simulink model "LIM_FOC_RNN_PID_1"  (R2021b)
settings: Solver=VariableStepAuto  StartTime=0.0  StopTime=3  RelTol=1e-3
values from neighbouring files (symbols this model uses):
  a1 = 1    [parameters_FOC.m]
  a2 = 1    [parameters_FOC.m]
  a3 = 1    [parameters_FOC.m]
  a4 = 1    [parameters_FOC.m]
  b1 = 1    [parameters_FOC.m]
  b2 = 1    [parameters_FOC.m]
  b3 = 1    [parameters_FOC.m]
  b4 = 1    [parameters_FOC.m]
  D = 0.25    [FOC_parameters_Basil.m]    (also in parameters_FOC.m)
  Llr = 0.005    [parameters_FOC.m]
  Lls = 0.005    [parameters_FOC.m]
  Lm = 0.0416    [FOC_parameters_Basil.m]    (also in parameters_FOC.m = 0.4)
  M = 4.775    [FOC_parameters_Basil.m]    (also in parameters_FOC.m)
  P = 2    [FOC_parameters_Basil.m]    (also in parameters_FOC.m = 4)
  ql = 1    [parameters_FOC.m]
  qq1 = 1    [parameters_FOC.m]
  qq2 = 1    [parameters_FOC.m]
  qq3 = 1    [parameters_FOC.m]
  qq4 = 1    [parameters_FOC.m]
  Rr = 11.78    [parameters_FOC.m]
  Rs = 13.2    [parameters_FOC.m]
  w1 = 1    [parameters_FOC.m]
  w2 = 1    [parameters_FOC.m]
  w3 = 1    [parameters_FOC.m]
  w4 = 1    [parameters_FOC.m]
libraries: neural x12, spsMosfetLib x6, slpidlib x3, spsVoltageMeasurementLib x3, simulink_extras x1, spsDCVoltageSourceLib x1, spsGroundLib x1, spspowerguiLib x1
settings Model: Creator=Hassan Alam  LastModifiedBy=Basilisk
settings SolverCC: ZeroCrossAlgorithm=Adaptive  AlgebraicLoopSolver=TrustRegion
settings DebuggingCC: MaskedZcDiagnostic=none  IgnoredZcDiagnostic=none  SFMachineParentedDataDiag=warning  ArithmeticOperatorsInVariantConditions=warning
settings SFSimCC: CustomCodeUndefinedFunction=UseInterfaceOnly

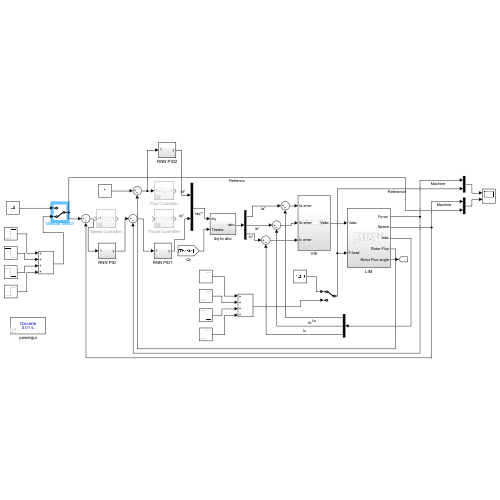
[thumbnail: Simulink's stored preview of the top-level diagram]
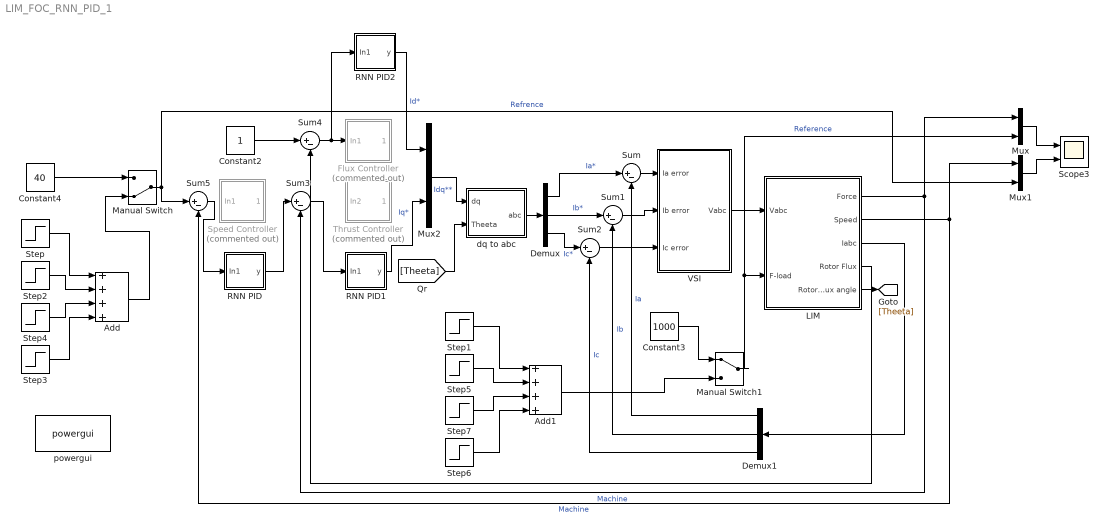
== system LIM_FOC_RNN_PID_1 ==
  Add : Sum  Inputs=++++
  Add1 : Sum  Inputs=++++
  Constant2 : Constant
  Constant3 : Constant  Value=1000
  Constant4 : Constant  Value=40
  Demux : Demux  Outputs=3
  Demux1 : Demux  Outputs=3
  Flux Controller : Subsystem  Commented=on
  LIM : Subsystem
  Manual Switch : ManualSwitch  CurrentSetting=0
  Manual Switch1 : ManualSwitch
  Mux : Mux  Inputs=2
  Mux1 : Mux  Inputs=2
  Mux2 : Mux  Inputs=2
  RNN PID : Subsystem
  RNN PID1 : Subsystem
  RNN PID2 : Subsystem
  Scope3 : Scope  NumInputPorts=2
  Speed Controller : Subsystem  Commented=on
  Step : Step  Time=0.5  Before=1  After=1.6  SampleTime=0
  Step1 : Step  Time=0.5  After=4  SampleTime=0
  Step2 : Step  Time=0.9  After=-0.4  SampleTime=0
  Step3 : Step  Time=2  After=0.5  SampleTime=0
  Step4 : Step  Time=1.5  After=-0.7  SampleTime=0
  Step5 : Step  Time=0.9  After=5  SampleTime=0
  Step6 : Step  Time=2  After=3  SampleTime=0
  Step7 : Step  Time=1.5  After=-2  SampleTime=0
  Sum{,1..5} (6 alike) : Sum  Inputs=|+-
  Thrust Controller : Subsystem  Commented=on
  VSI : Subsystem
  dq to abc : Subsystem
  powergui : spspowerguiLib/powergui  Priority=1  SimulationMode=Discrete  SampleTime=0.01  frequency=60  Iterations=50  frequencyindice=0  Pbase=100e6  ErrMax=1e-4  UnitsV=kV  UnitsW=MW  buscounter=0  FunctionMessages=off  echomessages=off  EnableUseOfTLC=off  CurrentSourceSwitches=off  DisableSnubberDevices=off  DisableRonSwitches=off  DisableVfSwitches=off  DisplayEquations=off  AutomaticDiscreteSolvers=off  SolverType=Tustin/Backward Euler (TBE)  Interpol=off  ExternalGateDelay=off  methode=off  Ts=100  x0status=blocks  SPID=on  SwTol=0  HookPort=off  NonlinearTolerance=1e-4  nMaxIteration=100  ContinueOnMaxIteration=off  RestoreLinks=warning  ResistiveCurrentMeasurement=off  Frange=[0:2:500]  Ylog=off  Xlog=on  ShowGrid=off  save=off  variable=ZData  structure=0  ZoomFFT=off  StartTime=0.0  cycles=1  DisplayStyle=1  fundamental=60  FreqAxis=off  MaxFrequency=1000  frequencyindicesteady=1  RmsSteady=1  display=off
  wires:
  Sum2/1 -> VSI/3(Ic error)
  Sum1/1 -> VSI/2(Ib error)
  Sum/1 -> VSI/1(Ia error)
  dq to abc/1(abc) -> Demux/1
  Demux/2 -> Sum1/1  "Ib*"
  Demux/1 -> Sum/1  "Ia*"
  Demux/3 -> Sum2/1  "Ic*"
  RNN PID1/1(y) -> Mux2/2  "Iq*"
  RNN PID2/1(y) -> Mux2/1  "Id*"
  Mux2/1 -> dq to abc/1(dq)  "Idq**"
  Demux1/1 -> Sum/2  "Ia"
  Demux1/2 -> Sum1/2  "Ib"
  Demux1/3 -> Sum2/2  "Ic"
  LIM/2(" Speed") -> Mux1/1, Sum5/2  "Machine"
  Constant2/1 -> Sum4/1
  Sum4/1 -> RNN PID2/1(In1), Flux Controller/1(In1)
  LIM/4(" Rotor Flux") -> Sum4/2
  [Theeta] -> dq to abc/2(Theeta)
  Constant4/1 -> Manual Switch/1
  VSI/1(Vabc) -> LIM/1(Vabc)
  Sum5/1 -> RNN PID/1(In1)
  LIM/5(" Rotor Flux angle") -> [Theeta]
  LIM/3(" Iabc") -> Demux1/1
  Sum3/1 -> RNN PID1/1(In1)
  Step/1 -> Add/1
  Constant3/1 -> Manual Switch1/1
  Manual Switch1/1 -> LIM/2(F-load), Mux/2  "Reference"
  Add1/1 -> Manual Switch1/2
  Manual Switch/1 -> Sum5/1, Mux1/2  "Refrence"
  Mux/1 -> Scope3/1
  Mux1/1 -> Scope3/2
  LIM/1("Force ") -> Mux/1, Sum3/2  "Machine"
  RNN PID/1(y) -> Sum3/1
  Step2/1 -> Add/2
  Step3/1 -> Add/4
  Step4/1 -> Add/3
  Add/1 -> Manual Switch/2
  Step7/1 -> Add1/3
  Step6/1 -> Add1/4
  Step5/1 -> Add1/2
  Step1/1 -> Add1/1

== system LIM_FOC_RNN_PID_1/Flux Controller ==
  In1 : Inport
  Gain2 : Gain  Gain=6000
  Gain3 : Gain  Gain=0.001
  Integrator : Integrator
  Sum2 : Sum
  Out1 : Outport
  wires:
  In1/1 -> Gain3/1, Gain2/1
  Gain3/1 -> Integrator/1
  Gain2/1 -> Sum2/1
  Integrator/1 -> Sum2/2
  Sum2/1 -> Out1/1

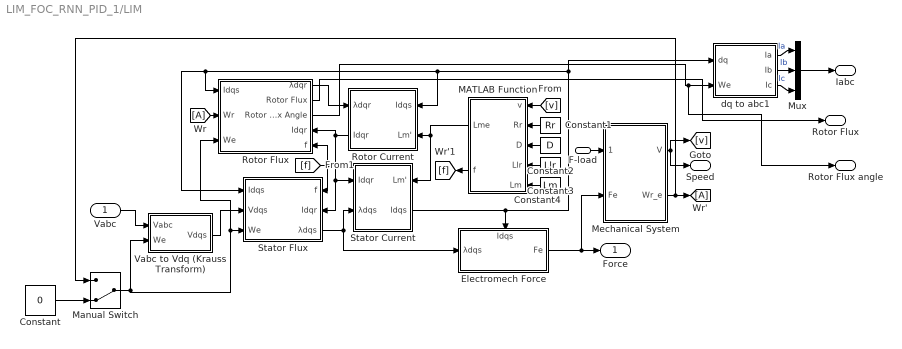
== system LIM_FOC_RNN_PID_1/LIM ==
  Vabc : Inport
  F-load : Inport  Port=2
  Constant : Constant  Value=0
  Constant1 : Constant  Value=Rr
  Constant2 : Constant  Value=D
  Constant3 : Constant  Value=Llr
  Constant4 : Constant  Value=Lm
  Electromech Force : Subsystem
      settings: PortSchema="{\"entries\":[{\"content\":{\"sides\":[{\"content\":{\"connectorIds\":[\"In1\"]},\"type\":\"ConnectorPlacement.EquallySpacedRectSide\",\"uuid\":\"a4b29cca-9cb0-4324-9244-2049ffc93668\"},{\"content\":{\"connectorIds\":[\"Out1\"],\"side\":\"RIGHT\"},\"type\":\"ConnectorPlacement.EquallySpacedRectSide\",\"uuid\":\"b20ff3ac-d40e-4f59-bb91-f6f2c0c6ca63\"},{\"content\":{\"connectorIds\":[\"In2\"],\"side\":\"TOP\"},\"type\":\"ConnectorPlacement.EquallySpacedRectSide\",\"uuid\":\"55342d43-b8f9-4aa9-846c-26670e92f4ca\"},{\"content\":{\"connectorIds\":[],\"side\":\"HIDDEN\"},\"type\":\"ConnectorPlacement.EquallySpacedRectSide\",\"uuid\":\"5fed22a0-a45a-430c-a997-0be85a9315bb\"}]},\"type\":\"ConnectorPlacement.EquallySpacedConnector\",\"uuid\":\"78d5652d-2b6b-4c50-974b-d09ad892483f\"}],\"packageUris\":[\"http://schema.mathworks.com/mf0/Connector/R2020b\"],\"version\":\"1.0\"}"
  MATLAB Function : MATLAB Function  TreatAsAtomicUnit=on
  Manual Switch : ManualSwitch  CurrentSetting=0
  Mechanical System : Subsystem
  Mux : Mux  Inputs=3
  Rotor Current : Subsystem
      settings: PortSchema="{\"entries\":[{\"content\":{\"sides\":[{\"content\":{\"connectorIds\":[\"In1\",\"Out1\"]},\"type\":\"ConnectorPlacement.EquallySpacedRectSide\",\"uuid\":\"b9a9f404-9b3b-4182-a50e-1bf7cef191e8\"},{\"content\":{\"connectorIds\":[\"In2\",\"In3\"],\"side\":\"RIGHT\"},\"type\":\"ConnectorPlacement.EquallySpacedRectSide\",\"uuid\":\"68159d79-7975-4fd0-98a3-7e35432781a2\"},{\"content\":{\"connectorIds\":[],\"side\":\"TOP\"},\"type\":\"ConnectorPlacement.EquallySpacedRectSide\",\"uuid\":\"0c4dbb5d-b4d4-4876-b829-49090bd6eeb8\"},{\"content\":{\"connectorIds\":[],\"side\":\"BOTTOM\"},\"type\":\"ConnectorPlacement.EquallySpacedRectSide\",\"uuid\":\"e42509db-2e5f-42f8-9a91-9046ba95e836\"},{\"content\":{\"connectorIds\":[],\"side\":\"HIDDEN\"},\"type\":\"ConnectorPlacement.EquallySpacedRectSide\",\"uuid\":\"f2a65973-682a-4dd6-b429-3fa72198cae4\"}]},\"type\":\"ConnectorPlacement.EquallySpacedConnector\",\"uuid\":\"744eb17f-cf6a-4151-90db-78263b57d619\"}],\"packageUris\":[\"http://schema.mathworks.com/mf0/Connector/R2020b\"],\"version\":\"1.0\"}"
  Rotor Flux : Subsystem
      settings: PortSchema="{\"entries\":[{\"content\":{\"sides\":[{\"content\":{\"connectorIds\":[\"In1\",\"In2\",\"In3\"]},\"type\":\"ConnectorPlacement.EquallySpacedRectSide\",\"uuid\":\"b9a9f404-9b3b-4182-a50e-1bf7cef191e8\"},{\"content\":{\"connectorIds\":[\"Out1\",\"Out2\",\"Out3\",\"In4\",\"In5\"],\"side\":\"RIGHT\"},\"type\":\"ConnectorPlacement.EquallySpacedRectSide\",\"uuid\":\"68159d79-7975-4fd0-98a3-7e35432781a2\"},{\"content\":{\"connectorIds\":[],\"side\":\"TOP\"},\"type\":\"ConnectorPlacement.EquallySpacedRectSide\",\"uuid\":\"0c4dbb5d-b4d4-4876-b829-49090bd6eeb8\"},{\"content\":{\"connectorIds\":[],\"side\":\"HIDDEN\"},\"type\":\"ConnectorPlacement.EquallySpacedRectSide\",\"uuid\":\"f2a65973-682a-4dd6-b429-3fa72198cae4\"}]},\"type\":\"ConnectorPlacement.EquallySpacedConnector\",\"uuid\":\"744eb17f-cf6a-4151-90db-78263b57d619\"}],\"packageUris\":[\"http://schema.mathworks.com/mf0/Connector/R2020b\"],\"version\":\"1.0\"}"
  Stator Current : Subsystem
      settings: PortSchema="{\"entries\":[{\"content\":{\"sides\":[{\"content\":{\"connectorIds\":[\"In1\",\"In2\"]},\"type\":\"ConnectorPlacement.EquallySpacedRectSide\",\"uuid\":\"c6a8d684-b7d2-4173-9e8a-0a77b360fa3b\"},{\"content\":{\"connectorIds\":[\"In3\",\"Out1\"],\"side\":\"RIGHT\"},\"type\":\"ConnectorPlacement.EquallySpacedRectSide\",\"uuid\":\"6b547613-238c-47a7-9a25-113e0bcf67e8\"},{\"content\":{\"connectorIds\":[],\"side\":\"TOP\"},\"type\":\"ConnectorPlacement.EquallySpacedRectSide\",\"uuid\":\"9eb731ca-d22d-4bff-90d4-9f452150afc4\"},{\"content\":{\"connectorIds\":[],\"side\":\"HIDDEN\"},\"type\":\"ConnectorPlacement.EquallySpacedRectSide\",\"uuid\":\"3386087c-4273-46bf-b0bc-9959c9fde15b\"}]},\"type\":\"ConnectorPlacement.EquallySpacedConnector\",\"uuid\":\"3fded039-aa6e-4722-8a98-01f4cd5eabc0\"}],\"packageUris\":[\"http://schema.mathworks.com/mf0/Connector/R2020b\"],\"version\":\"1.0\"}"
  Stator Flux : Subsystem
      settings: PortSchema="{\"entries\":[{\"content\":{\"sides\":[{\"content\":{\"connectorIds\":[\"In1\",\"In2\",\"In3\"]},\"type\":\"ConnectorPlacement.EquallySpacedRectSide\",\"uuid\":\"a4b29cca-9cb0-4324-9244-2049ffc93668\"},{\"content\":{\"connectorIds\":[\"In4\",\"In5\",\"Out1\"],\"side\":\"RIGHT\"},\"type\":\"ConnectorPlacement.EquallySpacedRectSide\",\"uuid\":\"b20ff3ac-d40e-4f59-bb91-f6f2c0c6ca63\"},{\"content\":{\"connectorIds\":[],\"side\":\"TOP\"},\"type\":\"ConnectorPlacement.EquallySpacedRectSide\",\"uuid\":\"55342d43-b8f9-4aa9-846c-26670e92f4ca\"},{\"content\":{\"connectorIds\":[],\"side\":\"HIDDEN\"},\"type\":\"ConnectorPlacement.EquallySpacedRectSide\",\"uuid\":\"5fed22a0-a45a-430c-a997-0be85a9315bb\"}]},\"type\":\"ConnectorPlacement.EquallySpacedConnector\",\"uuid\":\"78d5652d-2b6b-4c50-974b-d09ad892483f\"}],\"packageUris\":[\"http://schema.mathworks.com/mf0/Connector/R2020b\"],\"version\":\"1.0\"}"
  Vabc to Vdq (Krauss Transform) : Subsystem
  dq to abc1 : Subsystem
  "Force " : Outport
  " Speed" : Outport  Port=2
  " Iabc" : Outport  Port=3
  " Rotor Flux" : Outport  Port=4
  " Rotor Flux angle" : Outport  Port=5
  wires:
  Electromech Force/1(Fe) -> Mechanical System/2(Fe), "Force "/1
  F-load/1 -> Mechanical System/1(F-load)
  Mechanical System/1(V) -> " Speed"/1, [v]
  Stator Flux/1(λdqs) -> Stator Current/2(λdqs), Electromech Force/1(λdqs)
  Stator Current/1(Idqs) -> Electromech Force/2(Idqs), dq to abc1/1(dq), Rotor Flux/1(Idqs), Stator Flux/1(Idqs), Rotor Current/2(Idqs)
  Rotor Flux/1(λdqr) -> Rotor Current/1(λdqr)
  Rotor Current/1(Idqr) -> Rotor Flux/4(Idqr), Stator Flux/5(Idqr), Stator Current/1(Idqr)
  [A] -> Rotor Flux/2(Wr)
  Vabc/1 -> Vabc to Vdq (Krauss Transform)/1(Vabc)
  Vabc to Vdq (Krauss Transform)/1(Vdqs) -> Stator Flux/2(Vdqs)
  MATLAB Function/1(Lme) -> Stator Current/3(Lm'), Rotor Current/3(Lm')
  [v] -> MATLAB Function/1(v)
  Constant1/1 -> MATLAB Function/2(Rr)
  Constant2/1 -> MATLAB Function/3(D)
  Constant3/1 -> MATLAB Function/4(Llr)
  Constant4/1 -> MATLAB Function/5(Lm)
  MATLAB Function/2(f) -> [f]
  [f] -> Rotor Flux/5(f), Stator Flux/4(f)
  Mechanical System/2(Wr_e) -> Manual Switch/1, [A]
  Manual Switch/1 -> Vabc to Vdq (Krauss Transform)/2(We), Rotor Flux/3(We), Stator Flux/3(We)
  Constant/1 -> Manual Switch/2
  Mux/1 -> " Iabc"/1
  dq to abc1/2(Ib) -> Mux/2  "Ib"
  dq to abc1/3(Ic) -> Mux/3  "Ic"
  dq to abc1/1(Ia) -> Mux/1  "Ia"
  Rotor Flux/2(Rotor Flux) -> " Rotor Flux"/1
  Rotor Flux/3(Rotor Flux Angle) -> " Rotor Flux angle"/1, dq to abc1/2(We)

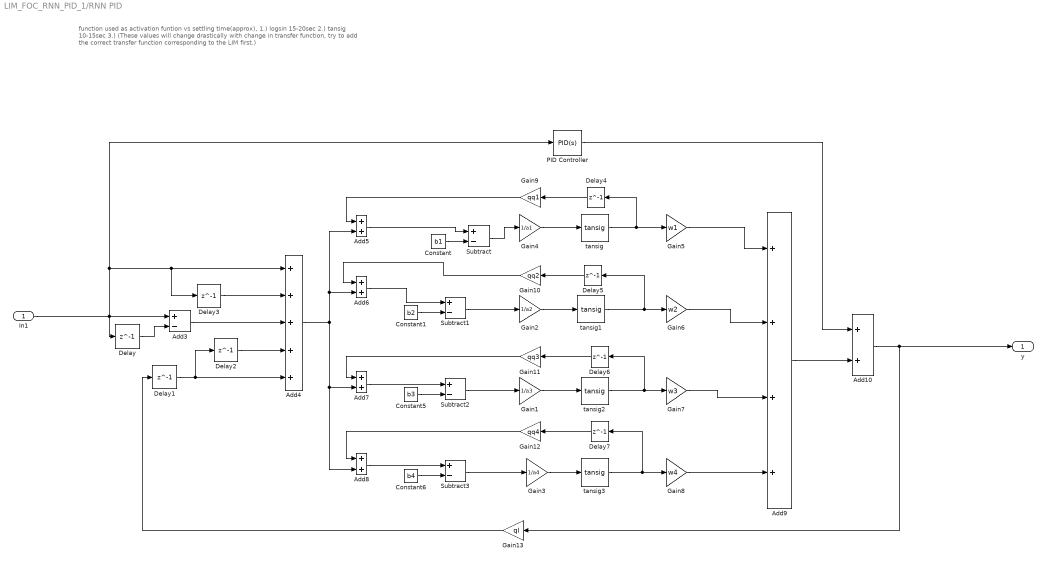
== system LIM_FOC_RNN_PID_1/RNN PID ==
  note: function used as activation funtion vs settling time(approx),
      | 1.) logsin   15-20sec
      | 2.) tansig   10-15sec
      | 3.)
      | (These values will change drastically with change in transfer function, try to add the correct transfer function corresponding to the LIM first.)
  In1 : Inport
  Add{5..8,10} (5 alike) : Sum
  Add3 : Sum  Inputs=+-
  Add4 : Sum  Inputs=+++++
  Add9 : Sum  Inputs=++++
  Constant : Constant  Value=b1
  Constant1 : Constant  Value=b2
  Constant5 : Constant  Value=b3
  Constant6 : Constant  Value=b4
  Delay{,1..7} (8 alike) : Delay  DelayLength=1
  Gain1 : Gain  Gain=1/a3
  Gain10 : Gain  Gain=qq2
  Gain11 : Gain  Gain=qq3
  Gain12 : Gain  Gain=qq4
  Gain13 : Gain  Gain=ql
  Gain2 : Gain  Gain=1/a2
  Gain3 : Gain  Gain=1/a4
  Gain4 : Gain  Gain=1/a1
  Gain5 : Gain  Gain=w1
  Gain6 : Gain  Gain=w2
  Gain7 : Gain  Gain=w3
  Gain8 : Gain  Gain=w4
  Gain9 : Gain  Gain=qq1
  PID Controller : slpidlib/PID Controller  Controller=PID  Form=Parallel  TimeDomain=Continuous-time  UseExternalTs=off  SampleTime=-1  IntegratorMethod=Forward Euler  FilterMethod=Forward Euler  ControllerParametersSource=internal  P=10  I=100  D=10  UseFilter=on  N=100  TunerSelectOption=Transfer Function Based (PID Tuner App)  InitialConditionSource=internal  InitialConditionForIntegrator=0  InitialConditionForFilter=0  DifferentiatorICPrevScaledInput=0  ExternalReset=none  TrackingMode=off  Kt=1  LimitOutput=off  SatLimitsSource=internal  UpperSaturationLimit=inf  LowerSaturationLimit=-inf  LinearizeAsGain=on  AntiWindupMode=none  Kb=1  POutMin=[]  POutMax=[]  IOutMin=[]  IOutMax=[]  DOutMin=[]  DOutMax=[]  NOutMin=[]  NOutMax=[]  SumOutMin=[]  SumOutMax=[]  SaturationOutMin=[]  SaturationOutMax=[]  PParamMin=[]  PParamMax=[]  IParamMin=[]  IParamMax=[]  DParamMin=[]  DParamMax=[]  NParamMin=[]  NParamMax=[]  KbParamMin=[]  KbParamMax=[]  KtParamMin=[]  KtParamMax=[]  KbOutMin=[]  KbOutMax=[]  KtOutMin=[]  KtOutMax=[]  IntegratorOutMin=[]  IntegratorOutMax=[]  FilterOutMin=[]  FilterOutMax=[]  SumI1OutMin=[]  SumI1OutMax=[]  SumI2OutMin=[]  SumI2OutMax=[]  SumI3OutMin=[]  SumI3OutMax=[]  SumI4OutMin=[]  SumI4OutMax=[]  SumDOutMin=[]  SumDOutMax=[]  DifferentiatorOutMin=[]  DifferentiatorOutMax=[]  FilterDiffOutCoefMin=[]  FilterDiffOutCoefMax=[]  ReciprocalOutMin=[]  ReciprocalOutMax=[]  SumDenOutMin=[]  SumDenOutMax=[]  SumNumOutMin=[]  SumNumOutMax=[]  DivideOutMin=[]  DivideOutMax=[]  UdiffTsProdOutMin=[]  UdiffTsProdOutMax=[]  NTsProdOutMin=[]  NTsProdOutMax=[]  UintegralTsProdOutMin=[]  UintegralTsProdOutMax=[]  UngainTsProdOutMin=[]  UngainTsProdOutMax=[]  IntegratorContinuousStateAttributes=''  IntegratorStateMustResolveToSignalObject=off  IntegratorRTWStateStorageClass=Auto  FilterContinuousStateAttributes=''  FilterStateMustResolveToSignalObject=off  FilterRTWStateStorageClass=Auto  ParallelPVariant=InternalParameters  IdealPVariant=Disabled  IVariant=InternalParameters  DVariant=InternalParameters  IntegratorVariant=Continuous  SatVariant=Disabled  AWVariant=Passthrough  PCopyVariant=Disabled  TRVariant=Disabled  FdbkBlocksVariant=Forward  IdealPFdbkVariant=Disabled  SatFdbkVariant=Disabled  DerivativeFilterVariant=ContFilter  NVariant=InternalParameters  NCopyVariant=Disabled  FilterICVariant=InternalICsFilter  IntegratorICVariant=InternalICs  ExternalResetVariant=Disabled  TRSumVariant=Passthrough  SumFdbkVariant=Disabled  SumVariant=Sum_PID  TsampFilterVariant=InternalTs  TsampNgainVariant=Passthrough  TsampIntegralVariant=Passthrough  ExternalSaturationOutDataTypeStr=Inherit: Same as second input
  Subtract{,1..3} (4 alike) : Sum  Inputs=+-
  tansig{,1..3} (4 alike) : neural/Transfer Functions/tansig
  y : Outport
  wires:
  Gain11/1 -> Add7/1
  Delay6/1 -> Gain11/1
  Constant5/1 -> Subtract2/2
  Gain8/1 -> Add9/4
  tansig1/1 -> Delay5/1, Gain6/1
  Gain1/1 -> tansig2/1
  tansig3/1 -> Delay7/1, Gain8/1
  Gain12/1 -> Add8/1
  Add10/1 -> y/1, Gain13/1
  Add3/1 -> Add4/3
  Delay/1 -> Add3/2
  Constant/1 -> Subtract/2
  Delay1/1 -> Delay2/1, Add4/5
  Add9/1 -> Add10/2
  Add5/1 -> Subtract/1
  Gain6/1 -> Add9/2
  Delay7/1 -> Gain12/1
  Subtract2/1 -> Gain1/1
  Gain7/1 -> Add9/3
  tansig2/1 -> Delay6/1, Gain7/1
  tansig/1 -> Delay4/1, Gain5/1
  Add4/1 -> Add8/2, Add7/2, Add6/2, Add5/2
  Gain5/1 -> Add9/1
  In1/1 -> PID Controller/1, Delay3/1, Add4/1, Add3/1, Delay/1
  Subtract3/1 -> Gain3/1
  Delay4/1 -> Gain9/1
  Gain4/1 -> tansig/1
  Add8/1 -> Subtract3/1
  Subtract/1 -> Gain4/1
  PID Controller/1 -> Add10/1
  Constant1/1 -> Subtract1/2
  Gain10/1 -> Add6/1
  Gain13/1 -> Delay1/1
  Gain9/1 -> Add5/1
  Constant6/1 -> Subtract3/2
  Delay2/1 -> Add4/4
  Add6/1 -> Subtract1/1
  Gain3/1 -> tansig3/1
  Gain2/1 -> tansig1/1
  Subtract1/1 -> Gain2/1
  Add7/1 -> Subtract2/1
  Delay3/1 -> Add4/2
  Delay5/1 -> Gain10/1

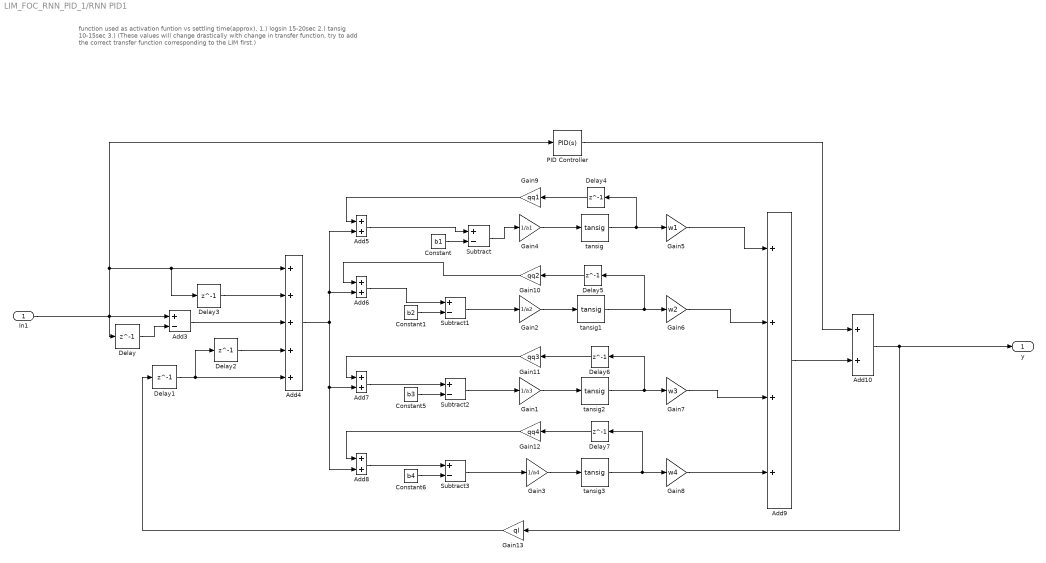
== system LIM_FOC_RNN_PID_1/RNN PID1 ==
  note: function used as activation funtion vs settling time(approx),
      | 1.) logsin   15-20sec
      | 2.) tansig   10-15sec
      | 3.)
      | (These values will change drastically with change in transfer function, try to add the correct transfer function corresponding to the LIM first.)
  In1 : Inport
  Add{5..8,10} (5 alike) : Sum
  Add3 : Sum  Inputs=+-
  Add4 : Sum  Inputs=+++++
  Add9 : Sum  Inputs=++++
  Constant : Constant  Value=b1
  Constant1 : Constant  Value=b2
  Constant5 : Constant  Value=b3
  Constant6 : Constant  Value=b4
  Delay{,1..7} (8 alike) : Delay  DelayLength=1
  Gain1 : Gain  Gain=1/a3
  Gain10 : Gain  Gain=qq2
  Gain11 : Gain  Gain=qq3
  Gain12 : Gain  Gain=qq4
  Gain13 : Gain  Gain=ql
  Gain2 : Gain  Gain=1/a2
  Gain3 : Gain  Gain=1/a4
  Gain4 : Gain  Gain=1/a1
  Gain5 : Gain  Gain=w1
  Gain6 : Gain  Gain=w2
  Gain7 : Gain  Gain=w3
  Gain8 : Gain  Gain=w4
  Gain9 : Gain  Gain=qq1
  PID Controller : slpidlib/PID Controller  Controller=PID  Form=Parallel  TimeDomain=Continuous-time  UseExternalTs=off  SampleTime=-1  IntegratorMethod=Forward Euler  FilterMethod=Forward Euler  ControllerParametersSource=internal  P=10  I=100  D=10  UseFilter=on  N=100  TunerSelectOption=Transfer Function Based (PID Tuner App)  InitialConditionSource=internal  InitialConditionForIntegrator=0  InitialConditionForFilter=0  DifferentiatorICPrevScaledInput=0  ExternalReset=none  TrackingMode=off  Kt=1  LimitOutput=off  SatLimitsSource=internal  UpperSaturationLimit=inf  LowerSaturationLimit=-inf  LinearizeAsGain=on  AntiWindupMode=none  Kb=1  POutMin=[]  POutMax=[]  IOutMin=[]  IOutMax=[]  DOutMin=[]  DOutMax=[]  NOutMin=[]  NOutMax=[]  SumOutMin=[]  SumOutMax=[]  SaturationOutMin=[]  SaturationOutMax=[]  PParamMin=[]  PParamMax=[]  IParamMin=[]  IParamMax=[]  DParamMin=[]  DParamMax=[]  NParamMin=[]  NParamMax=[]  KbParamMin=[]  KbParamMax=[]  KtParamMin=[]  KtParamMax=[]  KbOutMin=[]  KbOutMax=[]  KtOutMin=[]  KtOutMax=[]  IntegratorOutMin=[]  IntegratorOutMax=[]  FilterOutMin=[]  FilterOutMax=[]  SumI1OutMin=[]  SumI1OutMax=[]  SumI2OutMin=[]  SumI2OutMax=[]  SumI3OutMin=[]  SumI3OutMax=[]  SumI4OutMin=[]  SumI4OutMax=[]  SumDOutMin=[]  SumDOutMax=[]  DifferentiatorOutMin=[]  DifferentiatorOutMax=[]  FilterDiffOutCoefMin=[]  FilterDiffOutCoefMax=[]  ReciprocalOutMin=[]  ReciprocalOutMax=[]  SumDenOutMin=[]  SumDenOutMax=[]  SumNumOutMin=[]  SumNumOutMax=[]  DivideOutMin=[]  DivideOutMax=[]  UdiffTsProdOutMin=[]  UdiffTsProdOutMax=[]  NTsProdOutMin=[]  NTsProdOutMax=[]  UintegralTsProdOutMin=[]  UintegralTsProdOutMax=[]  UngainTsProdOutMin=[]  UngainTsProdOutMax=[]  IntegratorContinuousStateAttributes=''  IntegratorStateMustResolveToSignalObject=off  IntegratorRTWStateStorageClass=Auto  FilterContinuousStateAttributes=''  FilterStateMustResolveToSignalObject=off  FilterRTWStateStorageClass=Auto  ParallelPVariant=InternalParameters  IdealPVariant=Disabled  IVariant=InternalParameters  DVariant=InternalParameters  IntegratorVariant=Continuous  SatVariant=Disabled  AWVariant=Passthrough  PCopyVariant=Disabled  TRVariant=Disabled  FdbkBlocksVariant=Forward  IdealPFdbkVariant=Disabled  SatFdbkVariant=Disabled  DerivativeFilterVariant=ContFilter  NVariant=InternalParameters  NCopyVariant=Disabled  FilterICVariant=InternalICsFilter  IntegratorICVariant=InternalICs  ExternalResetVariant=Disabled  TRSumVariant=Passthrough  SumFdbkVariant=Disabled  SumVariant=Sum_PID  TsampFilterVariant=InternalTs  TsampNgainVariant=Passthrough  TsampIntegralVariant=Passthrough  ExternalSaturationOutDataTypeStr=Inherit: Same as second input
  Subtract{,1..3} (4 alike) : Sum  Inputs=+-
  tansig{,1..3} (4 alike) : neural/Transfer Functions/tansig
  y : Outport
  wires:
  Delay5/1 -> Gain10/1
  Delay3/1 -> Add4/2
  Add7/1 -> Subtract2/1
  Subtract1/1 -> Gain2/1
  Gain2/1 -> tansig1/1
  Gain3/1 -> tansig3/1
  Add6/1 -> Subtract1/1
  Delay2/1 -> Add4/4
  Constant6/1 -> Subtract3/2
  Gain9/1 -> Add5/1
  Gain13/1 -> Delay1/1
  Gain10/1 -> Add6/1
  Constant1/1 -> Subtract1/2
  PID Controller/1 -> Add10/1
  Subtract/1 -> Gain4/1
  Add8/1 -> Subtract3/1
  Gain4/1 -> tansig/1
  Delay4/1 -> Gain9/1
  Subtract3/1 -> Gain3/1
  In1/1 -> Delay/1, Add3/1, Add4/1, Delay3/1, PID Controller/1
  Gain5/1 -> Add9/1
  Add4/1 -> Add5/2, Add6/2, Add7/2, Add8/2
  tansig/1 -> Gain5/1, Delay4/1
  tansig2/1 -> Gain7/1, Delay6/1
  Gain7/1 -> Add9/3
  Subtract2/1 -> Gain1/1
  Delay7/1 -> Gain12/1
  Gain6/1 -> Add9/2
  Add5/1 -> Subtract/1
  Add9/1 -> Add10/2
  Delay1/1 -> Add4/5, Delay2/1
  Constant/1 -> Subtract/2
  Delay/1 -> Add3/2
  Add3/1 -> Add4/3
  Add10/1 -> Gain13/1, y/1
  Gain12/1 -> Add8/1
  tansig3/1 -> Gain8/1, Delay7/1
  Gain1/1 -> tansig2/1
  tansig1/1 -> Gain6/1, Delay5/1
  Gain8/1 -> Add9/4
  Constant5/1 -> Subtract2/2
  Delay6/1 -> Gain11/1
  Gain11/1 -> Add7/1

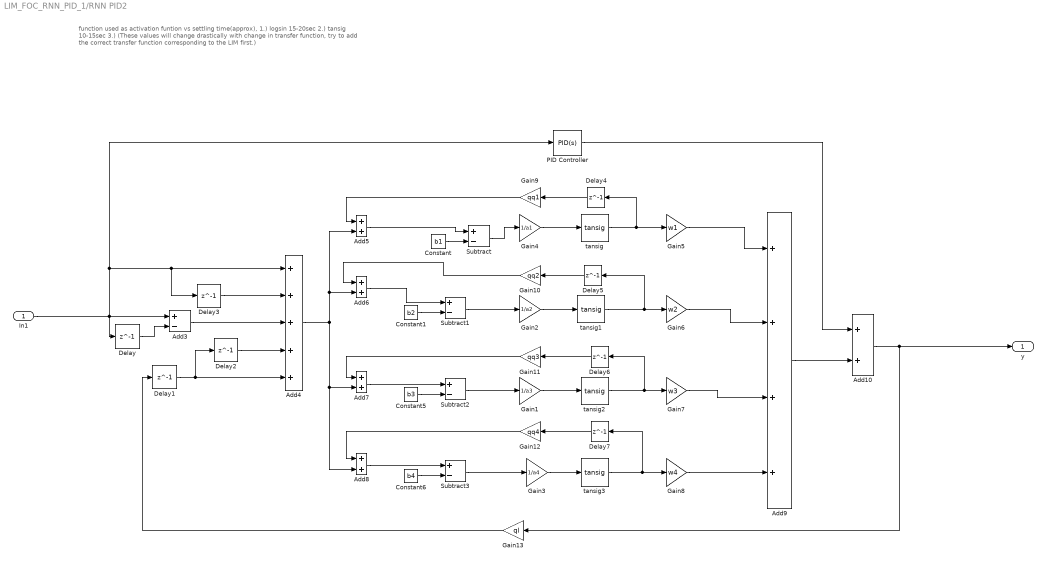
== system LIM_FOC_RNN_PID_1/RNN PID2 ==
  note: function used as activation funtion vs settling time(approx),
      | 1.) logsin   15-20sec
      | 2.) tansig   10-15sec
      | 3.)
      | (These values will change drastically with change in transfer function, try to add the correct transfer function corresponding to the LIM first.)
  In1 : Inport
  Add{5..8,10} (5 alike) : Sum
  Add3 : Sum  Inputs=+-
  Add4 : Sum  Inputs=+++++
  Add9 : Sum  Inputs=++++
  Constant : Constant  Value=b1
  Constant1 : Constant  Value=b2
  Constant5 : Constant  Value=b3
  Constant6 : Constant  Value=b4
  Delay{,1..7} (8 alike) : Delay  DelayLength=1
  Gain1 : Gain  Gain=1/a3
  Gain10 : Gain  Gain=qq2
  Gain11 : Gain  Gain=qq3
  Gain12 : Gain  Gain=qq4
  Gain13 : Gain  Gain=ql
  Gain2 : Gain  Gain=1/a2
  Gain3 : Gain  Gain=1/a4
  Gain4 : Gain  Gain=1/a1
  Gain5 : Gain  Gain=w1
  Gain6 : Gain  Gain=w2
  Gain7 : Gain  Gain=w3
  Gain8 : Gain  Gain=w4
  Gain9 : Gain  Gain=qq1
  PID Controller : slpidlib/PID Controller  Controller=PID  Form=Parallel  TimeDomain=Continuous-time  UseExternalTs=off  SampleTime=-1  IntegratorMethod=Forward Euler  FilterMethod=Forward Euler  ControllerParametersSource=internal  P=1  I=1  D=0  UseFilter=on  N=100  TunerSelectOption=Transfer Function Based (PID Tuner App)  InitialConditionSource=internal  InitialConditionForIntegrator=0  InitialConditionForFilter=0  DifferentiatorICPrevScaledInput=0  ExternalReset=none  TrackingMode=off  Kt=1  LimitOutput=off  SatLimitsSource=internal  UpperSaturationLimit=inf  LowerSaturationLimit=-inf  LinearizeAsGain=on  AntiWindupMode=none  Kb=1  POutMin=[]  POutMax=[]  IOutMin=[]  IOutMax=[]  DOutMin=[]  DOutMax=[]  NOutMin=[]  NOutMax=[]  SumOutMin=[]  SumOutMax=[]  SaturationOutMin=[]  SaturationOutMax=[]  PParamMin=[]  PParamMax=[]  IParamMin=[]  IParamMax=[]  DParamMin=[]  DParamMax=[]  NParamMin=[]  NParamMax=[]  KbParamMin=[]  KbParamMax=[]  KtParamMin=[]  KtParamMax=[]  KbOutMin=[]  KbOutMax=[]  KtOutMin=[]  KtOutMax=[]  IntegratorOutMin=[]  IntegratorOutMax=[]  FilterOutMin=[]  FilterOutMax=[]  SumI1OutMin=[]  SumI1OutMax=[]  SumI2OutMin=[]  SumI2OutMax=[]  SumI3OutMin=[]  SumI3OutMax=[]  SumI4OutMin=[]  SumI4OutMax=[]  SumDOutMin=[]  SumDOutMax=[]  DifferentiatorOutMin=[]  DifferentiatorOutMax=[]  FilterDiffOutCoefMin=[]  FilterDiffOutCoefMax=[]  ReciprocalOutMin=[]  ReciprocalOutMax=[]  SumDenOutMin=[]  SumDenOutMax=[]  SumNumOutMin=[]  SumNumOutMax=[]  DivideOutMin=[]  DivideOutMax=[]  UdiffTsProdOutMin=[]  UdiffTsProdOutMax=[]  NTsProdOutMin=[]  NTsProdOutMax=[]  UintegralTsProdOutMin=[]  UintegralTsProdOutMax=[]  UngainTsProdOutMin=[]  UngainTsProdOutMax=[]  IntegratorContinuousStateAttributes=''  IntegratorStateMustResolveToSignalObject=off  IntegratorRTWStateStorageClass=Auto  FilterContinuousStateAttributes=''  FilterStateMustResolveToSignalObject=off  FilterRTWStateStorageClass=Auto  ParallelPVariant=InternalParameters  IdealPVariant=Disabled  IVariant=InternalParameters  DVariant=InternalParameters  IntegratorVariant=Continuous  SatVariant=Disabled  AWVariant=Passthrough  PCopyVariant=Disabled  TRVariant=Disabled  FdbkBlocksVariant=Forward  IdealPFdbkVariant=Disabled  SatFdbkVariant=Disabled  DerivativeFilterVariant=ContFilter  NVariant=InternalParameters  NCopyVariant=Disabled  FilterICVariant=InternalICsFilter  IntegratorICVariant=InternalICs  ExternalResetVariant=Disabled  TRSumVariant=Passthrough  SumFdbkVariant=Disabled  SumVariant=Sum_PID  TsampFilterVariant=InternalTs  TsampNgainVariant=Passthrough  TsampIntegralVariant=Passthrough  ExternalSaturationOutDataTypeStr=Inherit: Same as second input
  Subtract{,1..3} (4 alike) : Sum  Inputs=+-
  tansig{,1..3} (4 alike) : neural/Transfer Functions/tansig
  y : Outport
  wires:
  Gain11/1 -> Add7/1
  Delay6/1 -> Gain11/1
  Constant5/1 -> Subtract2/2
  Gain8/1 -> Add9/4
  tansig1/1 -> Delay5/1, Gain6/1
  Gain1/1 -> tansig2/1
  tansig3/1 -> Delay7/1, Gain8/1
  Gain12/1 -> Add8/1
  Add10/1 -> y/1, Gain13/1
  Add3/1 -> Add4/3
  Delay/1 -> Add3/2
  Constant/1 -> Subtract/2
  Delay1/1 -> Delay2/1, Add4/5
  Add9/1 -> Add10/2
  Add5/1 -> Subtract/1
  Gain6/1 -> Add9/2
  Delay7/1 -> Gain12/1
  Subtract2/1 -> Gain1/1
  Gain7/1 -> Add9/3
  tansig2/1 -> Delay6/1, Gain7/1
  tansig/1 -> Delay4/1, Gain5/1
  Add4/1 -> Add8/2, Add7/2, Add6/2, Add5/2
  Gain5/1 -> Add9/1
  In1/1 -> PID Controller/1, Delay3/1, Add4/1, Add3/1, Delay/1
  Subtract3/1 -> Gain3/1
  Delay4/1 -> Gain9/1
  Gain4/1 -> tansig/1
  Add8/1 -> Subtract3/1
  Subtract/1 -> Gain4/1
  PID Controller/1 -> Add10/1
  Constant1/1 -> Subtract1/2
  Gain10/1 -> Add6/1
  Gain13/1 -> Delay1/1
  Gain9/1 -> Add5/1
  Constant6/1 -> Subtract3/2
  Delay2/1 -> Add4/4
  Add6/1 -> Subtract1/1
  Gain3/1 -> tansig3/1
  Gain2/1 -> tansig1/1
  Subtract1/1 -> Gain2/1
  Add7/1 -> Subtract2/1
  Delay3/1 -> Add4/2
  Delay5/1 -> Gain10/1

== system LIM_FOC_RNN_PID_1/Speed Controller ==
  In1 : Inport
  Add : Sum  Inputs=+++
  Derivative1 : Derivative
  Gain : Gain
  Gain1 : Gain  Gain=pi/t
  Gain4 : Gain  Gain=0.004
  Integrator1 : Integrator
  Kps : Gain  Gain=20
  Saturation : Saturate  UpperLimit=50  LowerLimit=-50
  Scope : Scope
  Out1 : Outport
  wires:
  Saturation/1 -> Out1/1, Scope/1
  Kps/1 -> Add/2
  Gain1/1 -> Gain/1, Gain4/1, Kps/1
  Gain/1 -> Integrator1/1
  Add/1 -> Saturation/1
  Integrator1/1 -> Add/1
  Derivative1/1 -> Add/3
  Gain4/1 -> Derivative1/1
  In1/1 -> Gain1/1

== system LIM_FOC_RNN_PID_1/Thrust Controller ==
  In2 : Inport
  Add : Sum
  Gain : Gain  Gain=0.09
  Integrator1 : Integrator
  Kps : Gain  Gain=12
  Scope : Scope
  Scope1 : Scope
  Out2 : Outport
  wires:
  In2/1 -> Scope/1, Gain/1, Kps/1
  Integrator1/1 -> Add/1
  Add/1 -> Scope1/1, Out2/1
  Kps/1 -> Add/2
  Gain/1 -> Integrator1/1

== system LIM_FOC_RNN_PID_1/VSI ==
  Ia error : Inport
  Ib error : Inport  Port=2
  Ic error : Inport  Port=3
  Mux : Mux  Inputs=3
  PWM Inverter : Subsystem
  Relay : Relay  OnSwitchValue=0.1  OffSwitchValue=-0.1
  Relay1 : Relay  OnSwitchValue=0.1  OffSwitchValue=-0.1
  Relay2 : Relay  OnSwitchValue=0.1  OffSwitchValue=-0.1
  Vabc : Outport
  wires:
  Ia error/1 -> Relay/1
  Ib error/1 -> Relay1/1
  Ic error/1 -> Relay2/1
  Relay1/1 -> PWM Inverter/2(Vb-Gate)
  Relay/1 -> PWM Inverter/1(Va-Gate)
  Relay2/1 -> PWM Inverter/3(Vc-Gate)
  PWM Inverter/2(Vb) -> Mux/2
  PWM Inverter/1(Va) -> Mux/1
  PWM Inverter/3(Vc) -> Mux/3
  Mux/1 -> Vabc/1

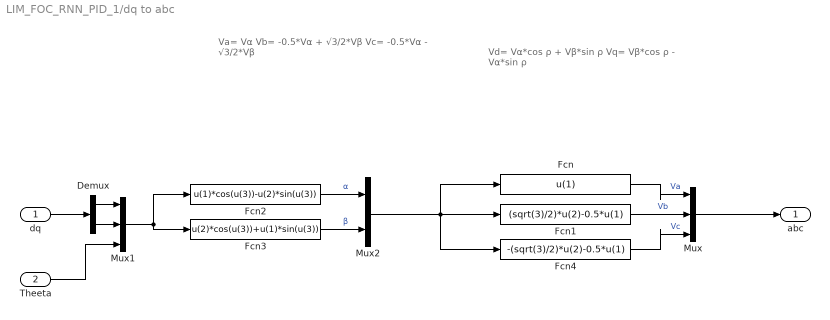
== system LIM_FOC_RNN_PID_1/dq to abc ==
  note: Va= Vα
      | Vb= -0.5*Vα + √3/2*Vβ
      | Vc= -0.5*Vα - √3/2*Vβ
  note: Vd= Vα*cos ρ + Vβ*sin ρ
      |
      | Vq= Vβ*cos ρ - Vα*sin ρ
  dq : Inport
  Theeta : Inport  Port=2
  Demux : Demux  Outputs=2
  Fcn : Fcn  Expr=u(1)
  Fcn1 : Fcn  Expr=(sqrt(3)/2)*u(2)-0.5*u(1)
  Fcn2 : Fcn  Expr=u(1)*cos(u(3))-u(2)*sin(u(3))
  Fcn3 : Fcn  Expr=u(2)*cos(u(3))+u(1)*sin(u(3))
  Fcn4 : Fcn  Expr=-(sqrt(3)/2)*u(2)-0.5*u(1)
  Mux : Mux  Inputs=3
  Mux1 : Mux  Inputs=3
  Mux2 : Mux  Inputs=2
  abc : Outport
  wires:
  Fcn/1 -> Mux/1  "Va"
  Fcn1/1 -> Mux/2  "Vb"
  Mux2/1 -> Fcn/1, Fcn4/1, Fcn1/1
  Fcn2/1 -> Mux2/1  "α"
  Fcn3/1 -> Mux2/2  "β"
  Theeta/1 -> Mux1/3
  Fcn4/1 -> Mux/3  "Vc"
  dq/1 -> Demux/1
  Mux1/1 -> Fcn3/1, Fcn2/1
  Demux/1 -> Mux1/1
  Demux/2 -> Mux1/2
  Mux/1 -> abc/1

== system LIM_FOC_RNN_PID_1/LIM/Electromech Force ==
  note: Fe=(3*pi/2*t)*(P/2)*[ λdsIqs-λqsIds]
  λdqs : Inport
  Idqs : Inport  Port=2
  Add : Sum  Inputs=+-
  Constant : Constant  Value=P
  Constant1 : Constant  Value=3/4
  Constant2 : Constant  Value=pi/t
  Demux : Demux  Outputs=2
  Demux1 : Demux  Outputs=2
  Product : Product  Inputs=4
  Product1 : Product
  Product2 : Product
  Fe : Outport
  wires:
  Product/1 -> Fe/1
  Constant1/1 -> Product/1
  Constant/1 -> Product/2
  λdqs/1 -> Demux/1
  Idqs/1 -> Demux1/1
  Add/1 -> Product/4
  Demux/1 -> Product1/1  "λds"
  Demux1/2 -> Product1/2  "Iqs"
  Demux/2 -> Product2/1  "λqs"
  Demux1/1 -> Product2/2  "Ids"
  Product1/1 -> Add/1
  Product2/1 -> Add/2
  Constant2/1 -> Product/3

== system LIM_FOC_RNN_PID_1/LIM/Mechanical System ==
  note: d/dt (v) = 1/M* [Fe-Fl-B*v]
  F-load : Inport
  Fe : Inport  Port=2
  Add : Sum  Inputs=+-
  Gain : Gain  Gain=P/2
  Gain1 : Gain  Gain=pi
  Gain2 : Gain  Gain=1/t
  Transfer Fcn : TransferFcn  Denominator=[M 0]
  V : Outport
  Wr_e : Outport  Port=2
  wires:
  Fe/1 -> Add/1
  F-load/1 -> Add/2
  Add/1 -> Transfer Fcn/1
  Gain2/1 -> Gain1/1
  Gain1/1 -> Wr_e/1
  Gain/1 -> Gain2/1, V/1
  Transfer Fcn/1 -> Gain/1

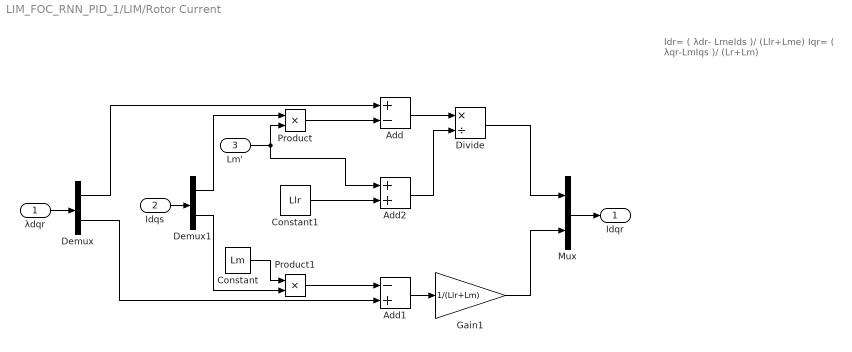
== system LIM_FOC_RNN_PID_1/LIM/Rotor Current ==
  note: Idr= ( λdr- LmeIds )/ (Llr+Lme)
      |
      | Iqr= ( λqr-LmIqs )/ (Lr+Lm)
  λdqr : Inport
  Idqs : Inport  Port=2
  Lm' : Inport  Port=3
  Add : Sum  Inputs=+-
  Add1 : Sum  Inputs=-+
  Add2 : Sum
  Constant : Constant  Value=Lm  VectorParams1D=off
  Constant1 : Constant  Value=Llr
  Demux : Demux  Outputs=2
  Demux1 : Demux  Outputs=2
  Divide : Product  Inputs=*/
  Gain1 : Gain  Gain=1/(Llr+Lm)
  Mux : Mux  Inputs=2
  Product : Product
  Product1 : Product
  Idqr : Outport
  wires:
  Mux/1 -> Idqr/1
  λdqr/1 -> Demux/1
  Idqs/1 -> Demux1/1
  Demux1/1 -> Product/1
  Demux1/2 -> Product1/2
  Demux/1 -> Add/1
  Demux/2 -> Add1/2
  Product/1 -> Add/2
  Product1/1 -> Add1/1
  Add/1 -> Divide/1
  Add1/1 -> Gain1/1
  Gain1/1 -> Mux/2
  Divide/1 -> Mux/1
  Constant/1 -> Product1/1
  Constant1/1 -> Add2/2
  Lm'/1 -> Add2/1, Product/2
  Add2/1 -> Divide/2

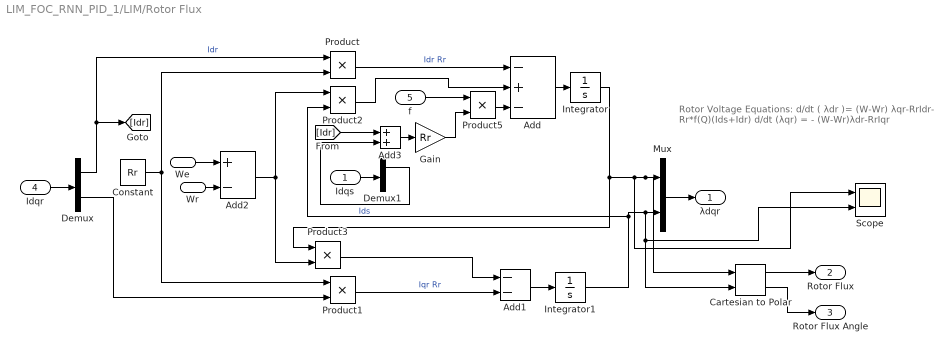
== system LIM_FOC_RNN_PID_1/LIM/Rotor Flux ==
  note: Rotor Voltage Equations:
      | d/dt ( λdr )= (W-Wr) λqr-RrIdr- Rr*f(Q)(Ids+Idr)
      | d/dt (λqr) = - (W-Wr)λdr-RrIqr
  Idqs : Inport
  Wr : Inport  Port=2
  We : Inport  Port=3
  Idqr : Inport  Port=4
  f : Inport  Port=5
  Add : Sum  Inputs=-+-
  Add1 : Sum  Inputs=--
  Add2 : Sum  Inputs=+-
  Add3 : Sum
  Cartesian to Polar : simulink_extras/Transformations/Cartesian to Polar
  Constant : Constant  Value=Rr
  Demux : Demux  Outputs=2
  Demux1 : Demux  Outputs=2
  Gain : Gain  Gain=Rr
  Integrator : Integrator
  Integrator1 : Integrator
  Mux : Mux  Inputs=2
  Product{,1..3,5} (5 alike) : Product
  Scope : Scope  NumInputPorts=2
  λdqr : Outport
  Rotor Flux : Outport  Port=2
  Rotor Flux Angle : Outport  Port=3
  wires:
  Mux/1 -> λdqr/1
  Idqr/1 -> Demux/1
  Demux/1 -> [Idr], Product/1  "Idr"
  Demux/2 -> Product1/2
  Constant/1 -> Product1/1, Product/2
  Product/1 -> Add/1  "Idr Rr"
  Product1/1 -> Add1/2  "Iqr Rr"
  Add/1 -> Integrator/1
  Add1/1 -> Integrator1/1
  We/1 -> Add2/1
  Wr/1 -> Add2/2
  Add2/1 -> Product3/2, Product2/1
  Product2/1 -> Add/2
  Product3/1 -> Add1/1
  Demux1/1 -> Add3/2  "Ids"
  Product5/1 -> Add/3
  Add3/1 -> Gain/1
  Gain/1 -> Product5/2
  f/1 -> Product5/1
  Idqs/1 -> Demux1/1
  [Idr] -> Add3/1
  Cartesian to Polar/1 -> Rotor Flux/1
  Cartesian to Polar/2 -> Rotor Flux Angle/1
  Integrator1/1 -> Scope/2, Cartesian to Polar/2, Mux/2, Product2/2
  Integrator/1 -> Product3/1, Scope/1, Cartesian to Polar/1, Mux/1

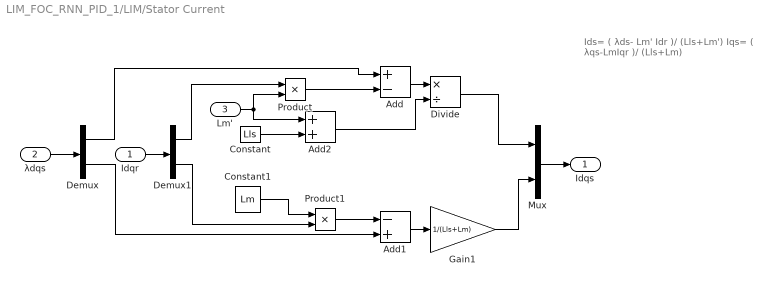
== system LIM_FOC_RNN_PID_1/LIM/Stator Current ==
  note: Ids= ( λds- Lm' Idr )/ (Lls+Lm')
      |
      | Iqs= ( λqs-LmIqr )/ (Lls+Lm)
  Idqr : Inport
  λdqs : Inport  Port=2
  Lm' : Inport  Port=3
  Add : Sum  Inputs=+-
  Add1 : Sum  Inputs=-+
  Add2 : Sum
  Constant : Constant  Value=Lls
  Constant1 : Constant  Value=Lm  VectorParams1D=off
  Demux : Demux  Outputs=2
  Demux1 : Demux  Outputs=2
  Divide : Product  Inputs=*/
  Gain1 : Gain  Gain=1/(Lls+Lm)
  Mux : Mux  Inputs=2
  Product : Product
  Product1 : Product
  Idqs : Outport
  wires:
  Demux/2 -> Add1/2
  Demux1/1 -> Product/1
  Product/1 -> Add/2
  Product1/1 -> Add1/1
  λdqs/1 -> Demux/1
  Add1/1 -> Gain1/1
  Mux/1 -> Idqs/1
  Idqr/1 -> Demux1/1
  Demux/1 -> Add/1
  Demux1/2 -> Product1/2
  Add/1 -> Divide/1
  Divide/1 -> Mux/1
  Gain1/1 -> Mux/2
  Constant1/1 -> Product1/1
  Lm'/1 -> Add2/1, Product/2
  Constant/1 -> Add2/2
  Add2/1 -> Divide/2

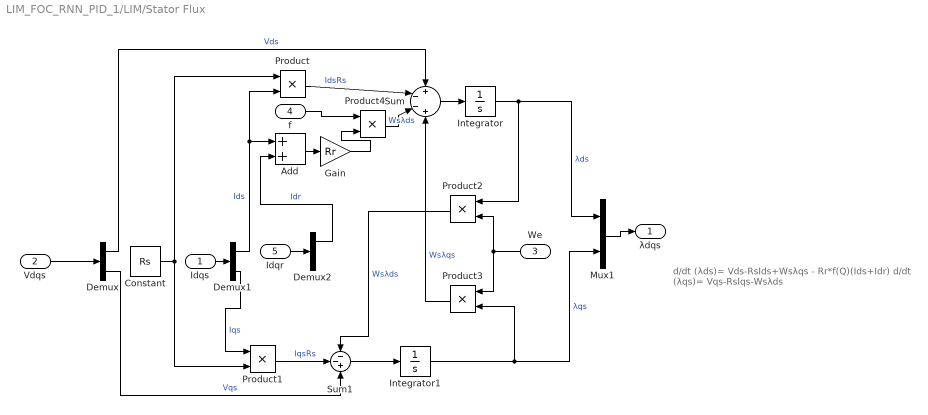
== system LIM_FOC_RNN_PID_1/LIM/Stator Flux ==
  note: d/dt (λds)= Vds-RsIds+Wsλqs - Rr*f(Q)(Ids+Idr)
      |
      | d/dt (λqs)= Vqs-RsIqs-Wsλds
  Idqs : Inport
  Vdqs : Inport  Port=2
  We : Inport  Port=3
  f : Inport  Port=4
  Idqr : Inport  Port=5
  Add : Sum
  Constant : Constant  Value=Rs
  Demux : Demux  Outputs=2
  Demux1 : Demux  Outputs=2
  Demux2 : Demux  Outputs=2
  Gain : Gain  Gain=Rr
  Integrator : Integrator
  Integrator1 : Integrator
  Mux1 : Mux  Inputs=2
  Product{,1..4} (5 alike) : Product
  Sum : Sum  Inputs=+--+
  Sum1 : Sum  Inputs=--+
  λdqs : Outport
  wires:
  Integrator1/1 -> Product3/2, Mux1/2  "λqs"
  Integrator/1 -> Product2/1, Mux1/1  "λds"
  Vdqs/1 -> Demux/1
  Idqs/1 -> Demux1/1
  Demux/1 -> Sum/1  "Vds"
  Sum/1 -> Integrator/1
  Constant/1 -> Product1/2, Product/1
  Demux1/1 -> Product/2, Add/1  "Ids"
  Product/1 -> Sum/2  "IdsRs"
  Sum1/1 -> Integrator1/1
  Demux/2 -> Sum1/3  "Vqs"
  Demux1/2 -> Product1/1  "Iqs"
  Product1/1 -> Sum1/2  "IqsRs"
  We/1 -> Product3/1, Product2/2
  Product3/1 -> Sum/4  "Wsλqs"
  Product2/1 -> Sum1/1  "Wsλds"
  Mux1/1 -> λdqs/1
  Idqr/1 -> Demux2/1
  Demux2/1 -> Add/2  "Idr"
  Add/1 -> Gain/1
  Gain/1 -> Product4/2
  Product4/1 -> Sum/3  "Wsλds"
  f/1 -> Product4/1

== system LIM_FOC_RNN_PID_1/LIM/Vabc to Vdq (Krauss Transform) ==
  note: Vα=2/3*[Va-0.5*{Vb+Vc}]
      |
      | Vβ=2/3*[√3/2 *{Vb-Vc}]
  note: Vd= Vα*cos ρ + Vβ*sin ρ
      |
      | Vq= Vβ*cos ρ - Vα*sin ρ
  Vabc : Inport
  We : Inport  Port=2
  Fcn : Fcn  Expr=(2/3)*(u(1)-0.5*u(2)-0.5*u(3))
  Fcn1 : Fcn  Expr=(2/3)*(sqrt(3)/2)*(u(2)-u(3))
  Fcn2 : Fcn  Expr=u(1)*cos(u(3))+u(2)*sin(u(3))
  Fcn3 : Fcn  Expr=u(2)*cos(u(3))-u(1)*sin(u(3))
  Integrator : Integrator
  Mux1 : Mux  Inputs=3
  Mux2 : Mux  Inputs=2
  Vdqs : Outport
  wires:
  Fcn/1 -> Mux1/1  "Vα"
  Fcn1/1 -> Mux1/2  "Vβ"
  Vabc/1 -> Fcn/1, Fcn1/1
  Mux2/1 -> Vdqs/1
  Integrator/1 -> Mux1/3
  Fcn2/1 -> Mux2/1  "Vd"
  Mux1/1 -> Fcn3/1, Fcn2/1
  Fcn3/1 -> Mux2/2  "Vq"
  We/1 -> Integrator/1

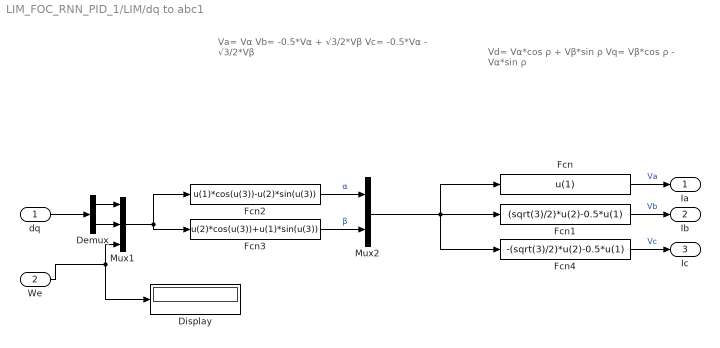
== system LIM_FOC_RNN_PID_1/LIM/dq to abc1 ==
  note: Vd= Vα*cos ρ + Vβ*sin ρ
      |
      | Vq= Vβ*cos ρ - Vα*sin ρ
  note: Va= Vα
      | Vb= -0.5*Vα + √3/2*Vβ
      | Vc= -0.5*Vα - √3/2*Vβ
  dq : Inport
  We : Inport  Port=2
  Demux : Demux  Outputs=2
  Display : Display
  Fcn : Fcn  Expr=u(1)
  Fcn1 : Fcn  Expr=(sqrt(3)/2)*u(2)-0.5*u(1)
  Fcn2 : Fcn  Expr=u(1)*cos(u(3))-u(2)*sin(u(3))
  Fcn3 : Fcn  Expr=u(2)*cos(u(3))+u(1)*sin(u(3))
  Fcn4 : Fcn  Expr=-(sqrt(3)/2)*u(2)-0.5*u(1)
  Mux1 : Mux  Inputs=3
  Mux2 : Mux  Inputs=2
  Ia : Outport
  Ib : Outport  Port=2
  Ic : Outport  Port=3
  wires:
  Demux/2 -> Mux1/2
  Demux/1 -> Mux1/1
  Mux1/1 -> Fcn2/1, Fcn3/1
  dq/1 -> Demux/1
  Fcn3/1 -> Mux2/2  "β"
  Fcn2/1 -> Mux2/1  "α"
  Mux2/1 -> Fcn1/1, Fcn4/1, Fcn/1
  Fcn/1 -> Ia/1  "Va"
  Fcn1/1 -> Ib/1  "Vb"
  Fcn4/1 -> Ic/1  "Vc"
  We/1 -> Mux1/3, Display/1

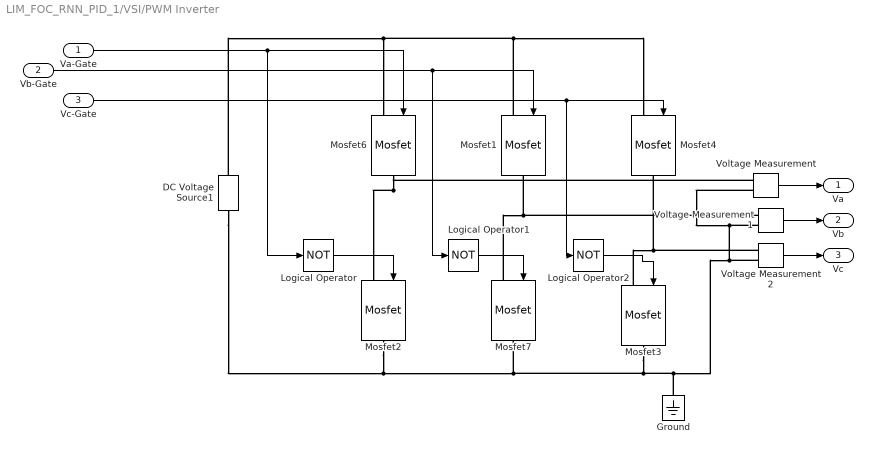
== system LIM_FOC_RNN_PID_1/VSI/PWM Inverter ==
  Va-Gate : Inport
  Vb-Gate : Inport  Port=2
  Vc-Gate : Inport  Port=3
  DC Voltage Source1 : spsDCVoltageSourceLib/DC Voltage Source  Amplitude=400  Measurements=None
  Ground : spsGroundLib/Ground  LConnTagsString=a
  Logical Operator : Logic  Operator=NOT  AllPortsSameDT=off  OutDataTypeStr=boolean
  Logical Operator1 : Logic  Operator=NOT  AllPortsSameDT=off  OutDataTypeStr=boolean
  Logical Operator2 : Logic  Operator=NOT  AllPortsSameDT=off  OutDataTypeStr=boolean
  Mosfet{1..4,6..7} (6 alike) : spsMosfetLib/Mosfet  Ron=0.1  Lon=0  Rd=0.01  Vfd=0  IC=0  Rs=1e5  Cs=inf  Measurements=off
  Voltage Measurement : spsVoltageMeasurementLib/Voltage Measurement  PhasorSimulation=off  OutputType=Complex  PSBequivalent=0
  Voltage Measurement1 : spsVoltageMeasurementLib/Voltage Measurement  PhasorSimulation=off  OutputType=Complex  PSBequivalent=0
  Voltage Measurement2 : spsVoltageMeasurementLib/Voltage Measurement  PhasorSimulation=off  OutputType=Complex  PSBequivalent=0
  Va : Outport
  Vb : Outport  Port=2
  Vc : Outport  Port=3
  wires:
  Voltage Measurement/1 -> Va/1
  Logical Operator1/1 -> Mosfet7/1
  Logical Operator/1 -> Mosfet2/1
  Voltage Measurement1/1 -> Vb/1
  Voltage Measurement2/1 -> Vc/1
  Logical Operator2/1 -> Mosfet3/1
  Vc-Gate/1 -> Mosfet4/1, Logical Operator2/1
  Vb-Gate/1 -> Mosfet1/1, Logical Operator1/1
  Va-Gate/1 -> Mosfet6/1, Logical Operator/1
  connections:
  Mosfet4/LConn1 -- Mosfet1/LConn1 -- DC Voltage Source1/RConn1 -- Mosfet6/LConn1
  Mosfet1/RConn1 -- Voltage Measurement1/LConn1 -- Mosfet7/LConn1
  Mosfet6/RConn1 -- Voltage Measurement/LConn1 -- Mosfet2/LConn1
  Mosfet4/RConn1 -- Voltage Measurement2/LConn1 -- Mosfet3/LConn1
  DC Voltage Source1/LConn1 -- Mosfet2/RConn1 -- Mosfet7/RConn1 -- Mosfet3/RConn1 -- Ground/LConn1 -- Voltage Measurement2/LConn2 -- Voltage Measurement1/LConn2 -- Voltage Measurement/LConn2

== matlab function LIM_FOC_RNN_PID_1/LIM/MATLAB Function ==
  data: v input; Lme output; Rr input; D input; Llr input; Lm input; f output
function [Lme,f]= fcn(v, Rr,D,Llr,Lm)
Q=abs((D*Rr)/(Llr*v));
f=(1-(exp(-Q)))/Q;
Lme = Lm*(1-f)
